simulink subsystem "InputFiltering"  (R2019b)
settings: Solver=VariableStepAuto  StartTime=0.0  StopTime=10.0  RelTol=1e-3
undefined symbols (not defined in the file): __PRM__SERIALIZED__DATA__, SubsystemReferenceBlock
libraries: FunctionCallDivider x1
settings Model: Creator=Nick  LastModifiedBy=Nick

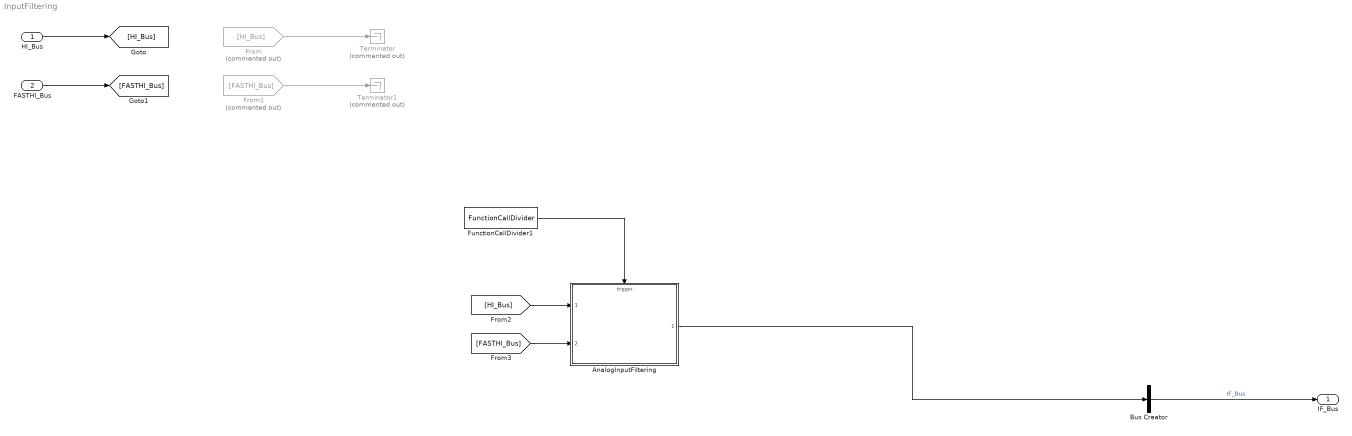
== system InputFiltering ==
  HI_Bus : Inport
  FASTHI_Bus : Inport  Port=2
  AnalogInputFiltering : Subsystem  BlockKeywords=__PRM__SERIALIZED__DATA__:SubsystemReferenceBlock  ReferencedSubsystem=AnalogInputFiltering
  Bus Creator : BusCreator  Inputs=1
  From : From  Commented=on  GotoTag=HI_Bus
  From1 : From  Commented=on  GotoTag=FASTHI_Bus
  FunctionCallDivider1 : FunctionCallDivider/Algroithms/FunctionCallDivider  counts=1
  Terminator : Terminator  Commented=on
  Terminator1 : Terminator  Commented=on
  IF_Bus : Outport
  wires:
  Bus Creator/1 -> IF_Bus/1  "IF_Bus"
  HI_Bus/1 -> [HI_Bus]
  From/1 -> Terminator/1
  From1/1 -> Terminator1/1
  FASTHI_Bus/1 -> [FASTHI_Bus]
  FunctionCallDivider1/1 -> AnalogInputFiltering/Trigger
  [FASTHI_Bus] -> AnalogInputFiltering/2
  [HI_Bus] -> AnalogInputFiltering/1
  AnalogInputFiltering/1 -> Bus Creator/1
